simulink model "PV_SUBSYSTEM"  (R2026a)
settings: Solver=VariableStepAuto
settings Model: Creator=S.THANUJ  LastModifiedBy=S.THANUJ

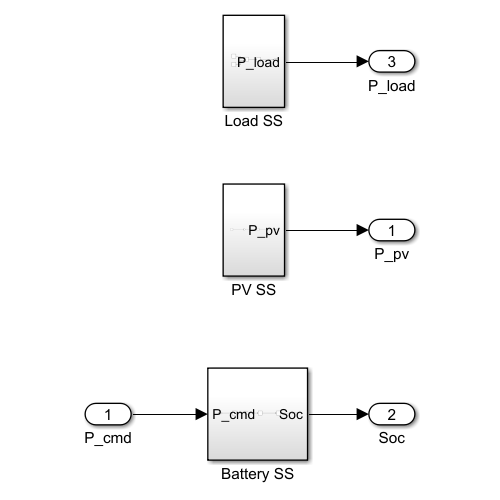
[thumbnail: Simulink's stored preview of the top-level diagram]
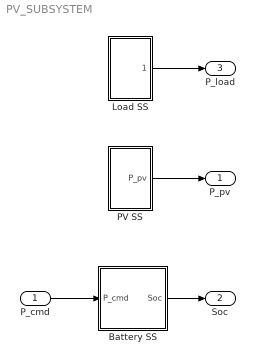
== system PV_SUBSYSTEM ==
  P_cmd : Inport
  Battery SS : Subsystem
  Load SS : Subsystem
  PV SS : Subsystem
  P_pv : Outport
  Soc : Outport  Port=2
  P_load : Outport  Port=3
  wires:
  PV SS/1(P_pv) -> P_pv/1
  P_cmd/1 -> Battery SS/1(P_cmd)
  Battery SS/1(Soc) -> Soc/1
  Load SS/1(P_load) -> P_load/1

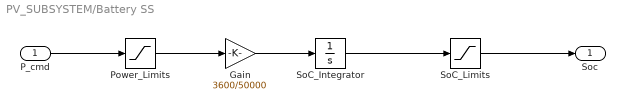
== system PV_SUBSYSTEM/Battery SS ==
  P_cmd : Inport
  Gain : Gain  Gain=3600/50000
  Power_Limits : Saturate  UpperLimit=5  LowerLimit=5
  SoC_Integrator : Integrator  InitialCondition=0.5
  SoC_Limits : Saturate  UpperLimit=0.9  LowerLimit=0.2
  Soc : Outport
  wires:
  Gain/1 -> SoC_Integrator/1
  SoC_Integrator/1 -> SoC_Limits/1
  Power_Limits/1 -> Gain/1
  P_cmd/1 -> Power_Limits/1
  SoC_Limits/1 -> Soc/1

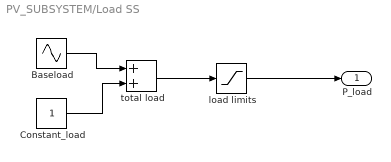
== system PV_SUBSYSTEM/Load SS ==
  Baseload : Sin  Amplitude=2  SampleTime=0
  Constant_load : Constant
  load limits : Saturate  UpperLimit=inf  LowerLimit=0.5
  total load : Sum
  P_load : Outport
  wires:
  Baseload/1 -> total load/1
  Constant_load/1 -> total load/2
  load limits/1 -> P_load/1
  total load/1 -> load limits/1

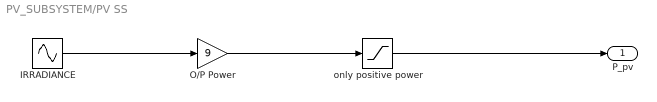
== system PV_SUBSYSTEM/PV SS ==
  IRRADIANCE : Sin  Amplitude=500  Bias=500  Frequency=2*pi/86400  SampleTime=0
  O/P Power : Gain  Gain=9
  only positive power : Saturate  UpperLimit=inf  LowerLimit=0
  P_pv : Outport
  wires:
  IRRADIANCE/1 -> O/P Power/1
  O/P Power/1 -> only positive power/1
  only positive power/1 -> P_pv/1
